simulink model "representacionBloquesED"  (R2026a)
settings: Solver=VariableStepAuto
InitFcn:
  | ip = 0.0079;
  | mc = 0.7031;
  | lp = 0.3302;
  | mp = 0.23;
  | fc = 0;
  | beq = 4.3;
  | g = 9.81;
  | bp = 0.0024;

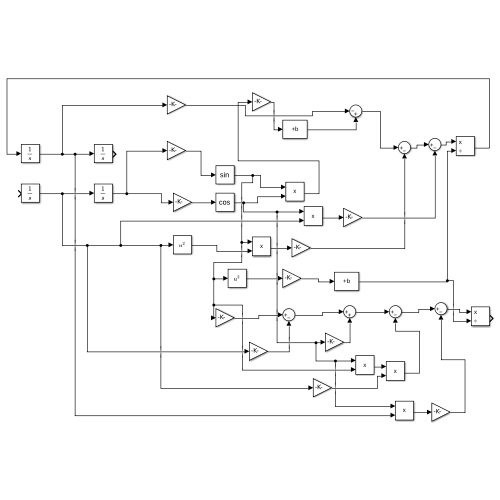
[thumbnail: Simulink's stored preview of the top-level diagram]
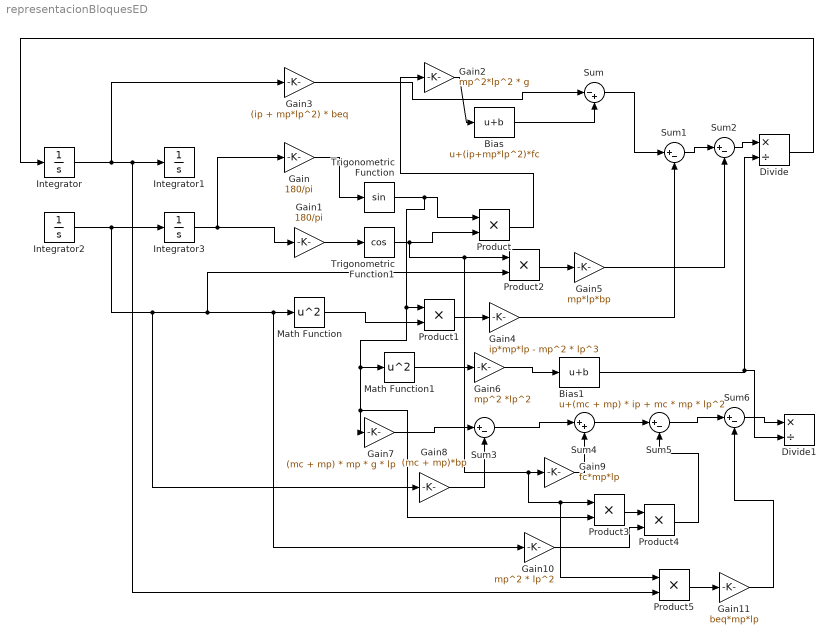
== system representacionBloquesED ==
  Bias : Bias  Bias=(ip+mp*lp^2)*fc  SaturateOnIntegerOverflow=off
  Bias1 : Bias  Bias=(mc + mp) * ip + mc * mp * lp^2  SaturateOnIntegerOverflow=off
  Divide : Product  Inputs=*/
  Divide1 : Product  Inputs=*/
  Gain : Gain  Gain=180/pi
  Gain1 : Gain  Gain=180/pi
  Gain10 : Gain  Gain=mp^2 * lp^2
  Gain11 : Gain  Gain=beq*mp*lp
  Gain2 : Gain  Gain=mp^2*lp^2 * g
  Gain3 : Gain  Gain=(ip + mp*lp^2) * beq
  Gain4 : Gain  Gain=ip*mp*lp - mp^2 * lp^3
  Gain5 : Gain  Gain=mp*lp*bp
  Gain6 : Gain  Gain=mp^2 *lp^2
  Gain7 : Gain  Gain=(mc + mp) * mp * g * lp
  Gain8 : Gain  Gain=(mc + mp)*bp
  Gain9 : Gain  Gain=fc*mp*lp
  Integrator{,1..3} (4 alike) : Integrator
  Math Function : Math  Operator=square
  Math Function1 : Math  Operator=square
  Product{,1..5} (6 alike) : Product
  Sum : Sum  Inputs=|-+
  Sum{1..3,5..6} (5 alike) : Sum  Inputs=|+-
  Sum4 : Sum  Inputs=|++
  Trigonometric Function : Trigonometry
  Trigonometric Function1 : Trigonometry  Operator=cos
  wires:
  Integrator/1 -> Product5/2, Integrator1/1, Gain3/1
  Integrator3/1 -> Gain1/1, Gain/1
  Trigonometric Function1/1 -> Product/2, Product5/1, Product3/1, Gain9/1, Product2/1
  Gain/1 -> Trigonometric Function/1
  Gain1/1 -> Trigonometric Function1/1
  Trigonometric Function/1 -> Product3/2, Gain7/1, Math Function1/1, Product1/1, Product/1
  Product/1 -> Gain2/1
  Gain2/1 -> Bias/1
  Bias/1 -> Sum/2
  Gain3/1 -> Sum/1
  Math Function/1 -> Product1/2
  Product1/1 -> Gain4/1
  Gain4/1 -> Sum1/2
  Sum/1 -> Sum1/1
  Sum1/1 -> Sum2/1
  Product2/1 -> Gain5/1
  Gain5/1 -> Sum2/2
  Sum2/1 -> Divide/1
  Math Function1/1 -> Gain6/1
  Gain6/1 -> Bias1/1
  Bias1/1 -> Divide1/2, Divide/2
  Divide/1 -> Integrator/1
  Gain7/1 -> Sum3/1
  Gain8/1 -> Sum3/2
  Sum3/1 -> Sum4/1
  Gain9/1 -> Sum4/2
  Sum4/1 -> Sum5/1
  Product4/1 -> Sum5/2
  Product3/1 -> Product4/1
  Gain10/1 -> Product4/2
  Integrator2/1 -> Gain8/1, Product2/2, Gain10/1, Math Function/1, Integrator3/1
  Sum5/1 -> Sum6/1
  Product5/1 -> Gain11/1
  Gain11/1 -> Sum6/2
  Sum6/1 -> Divide1/1
